simulink model "QPSK1"  (Simulink 8.2)
settings: Solver=ode45  StartTime=0.0  StopTime=10  MaxStep=0.00001  MinStep=0.000005  RelTol=1e-3
libraries: visionconversions x2, simulink_extras x2, dspsigops x2, commchan3 x1, commrandsrc2 x1, commsink2 x1, dspswit3 x1
settings Model: Creator=Yi_Liu  LastModifiedBy=Yi_Liu
settings DataIOCC: SignalLoggingSaveFormat=Dataset
settings OptimizationCC: ExpressionDepthLimit=128
settings DebuggingCC: FcnCallInpInsideContextMsg=EnableAllAsError  StateNameClashWarn=none
settings GRTTargetCC: CombineOutputUpdateFcns=on  GRTInterface=off

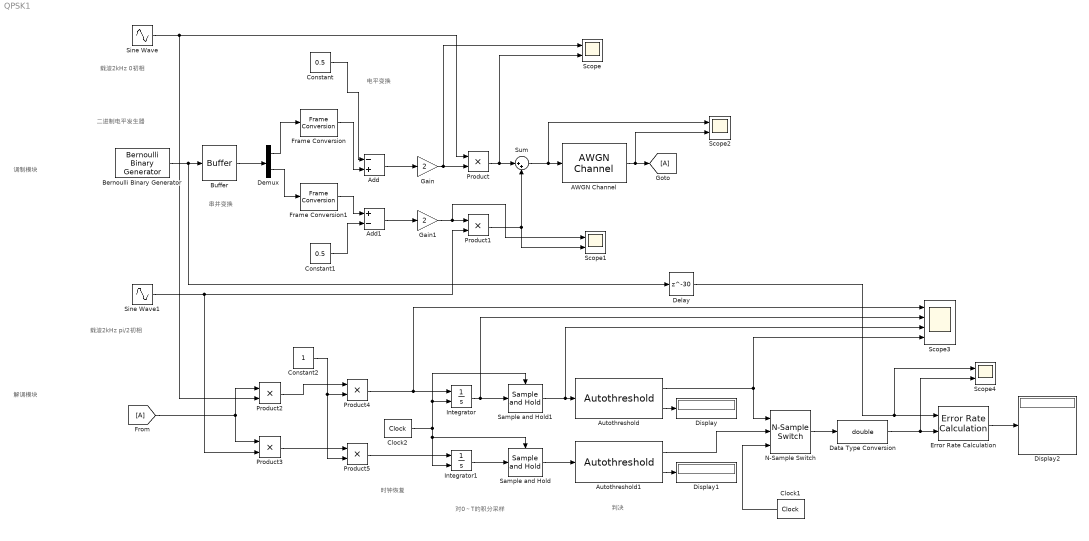
== system QPSK1 ==
  note: 判决
  note: 对0～T的积分采样
  note: 时钟恢复
  note: 调制模块
  note: 电平变换
  note: 串并变换
  note: 载波2kHz 0初相
  note: 二进制电平发生器
  note: 载波2kHz pi/2初相
  note: 解调模块
  AWGN Channel : commchan3/AWGN Channel  InputProcessing=Columns as channels (frame based)  seed=128  noiseMode=Variance from mask  EbNodB=10  EsNodB=10  SNRdB=10  bitsPerSym=1  Ps=1  Tsym=1  variance=0.01
  Add : Sum  Inputs=-+
  Add1 : Sum  Inputs=+-
  Autothreshold : visionconversions/Autothreshold  operator=>  threshOut=on  effMetricOut=off  userDefinedRange=off  umin=0  umax=255  outOfRngOpt=Warn and saturate  scaleThreshold=off  scaleFactor=1  P1Mode=Specify word length  P1WordLength=32  P1FracLength=30  P2Mode=Specify word length  P2WordLength=32  P2FracLength=22  P3Mode=Specify word length  P3WordLength=32  P3FracLength=14  P4Mode=Binary point scaling  P4WordLength=32  P4FracLength=15  Q1Mode=Specify word length  Q1WordLength=32  Q1FracLength=16  EMMode=Specify word length  EMWordLength=16  EMFracLength=14  roundingMode=Floor  overflowMode=off
  Autothreshold1 : visionconversions/Autothreshold  operator=>  threshOut=on  effMetricOut=off  userDefinedRange=off  umin=0  umax=255  outOfRngOpt=Warn and saturate  scaleThreshold=off  scaleFactor=1  P1Mode=Specify word length  P1WordLength=32  P1FracLength=30  P2Mode=Specify word length  P2WordLength=32  P2FracLength=22  P3Mode=Specify word length  P3WordLength=32  P3FracLength=14  P4Mode=Binary point scaling  P4WordLength=32  P4FracLength=15  Q1Mode=Specify word length  Q1WordLength=32  Q1FracLength=16  EMMode=Specify word length  EMWordLength=16  EMFracLength=14  roundingMode=Floor  overflowMode=off
  Bernoulli Binary Generator : commrandsrc2/Bernoulli Binary Generator  P=0.5  seed=64  Ts=0.001  frameBased=off  sampPerFrame=1  orient=off  outDataType=double
  Buffer : Buffer  N=2  TreatMby1Signals=One channel
  Clock1 : simulink_extras/Flip Flops/Clock  period=0.002
  Clock2 : simulink_extras/Flip Flops/Clock  period=0.002
  Constant : Constant  Value=0.5
  Constant1 : Constant  Value=0.5
  Constant2 : Constant
  Data Type Conversion : DataTypeConversion  OutDataTypeStr=double
  Delay : Delay  DelayLength=30  InitialCondition=0  SampleTime=0.0001
  Demux : Demux  Outputs=2
  Display : Display
  Display1 : Display
  Display2 : Display
  Error Rate Calculation : commsink2/Error Rate Calculation  N=0  st_delay=0  cp_mode=Entire frame  subframe=[]  PMode=Port  WsName=ErrorVec  RsMode2=off  stop=off  numErr=100  maxBits=1e6
  Frame Conversion : FrameConversion  OutFrame=Sample-based
  Frame Conversion1 : FrameConversion  OutFrame=Sample-based
  Gain : Gain  Gain=2
  Gain1 : Gain  Gain=2
  Integrator : Integrator  ExternalReset=rising
  Integrator1 : Integrator  ExternalReset=rising
  N-Sample Switch : dspswit3/N-Sample Switch  N=1  reset=on  TriggerType=Falling edge  Ts=-1
  Product{,1..5} (6 alike) : Product
  Sample and Hold : dspsigops/Sample and Hold  trig=Falling edge  initCond=0  latchinput=off
  Sample and Hold1 : dspsigops/Sample and Hold  trig=Falling edge  initCond=0  latchinput=off
  Scope{,1..2,4} (4 alike) : Scope  NumInputPorts=2
      Scope settings: YMin=-2~-2  YMax=2~2
      Scope1 settings: YMin=-2~-2  YMax=2~2
      Scope2 settings: YMin=-2~-2  YMax=2~2  SaveName=ScopeData2
      Scope4 settings: YMin=-2~-2  YMax=2~2  SaveName=ScopeData4
  Scope3 : Scope  NumInputPorts=4
      settings: YMin=-2~-2~-5~-5  YMax=2~2~5~5  SaveName=ScopeData3
  Sine Wave : Sin  Frequency=2*pi*2000  SampleTime=0
  Sine Wave1 : Sin  Frequency=2*pi*2000  Phase=pi/2  SampleTime=0
  Sum : Sum  Inputs=|++
  wires:
  Buffer/1 -> Demux/1
  Demux/1 -> Frame Conversion/1
  Demux/2 -> Frame Conversion1/1
  Add/1 -> Gain/1
  Frame Conversion1/1 -> Add1/1
  Frame Conversion/1 -> Add/2
  Constant/1 -> Add/1
  Constant1/1 -> Add1/2
  Add1/1 -> Gain1/1
  Gain1/1 -> Scope1/1, Product1/1
  Gain/1 -> Scope/1, Product/2
  Sine Wave1/1 -> Product1/2, Product3/2
  Sine Wave/1 -> Product2/2, Product/1
  Product1/1 -> Sum/2, Scope1/2
  Sum/1 -> Scope2/1, AWGN Channel/1
  AWGN Channel/1 -> Scope2/2, [A]
  Product3/1 -> Product5/1
  Constant2/1 -> Product4/2, Product5/2
  Clock2/1 -> Sample and Hold/Trigger, Integrator1/2, Integrator/2, Sample and Hold1/Trigger
  Product4/1 -> Scope3/1, Integrator/1
  Product5/1 -> Integrator1/1
  Autothreshold/1 -> Scope3/4, N-Sample Switch/1
  Autothreshold1/1 -> N-Sample Switch/2
  Clock1/1 -> N-Sample Switch/3
  Autothreshold/2 -> Display/1
  Autothreshold1/2 -> Display1/1
  [A] -> Product3/1, Product2/1
  Error Rate Calculation/1 -> Display2/1
  Product2/1 -> Product4/1
  Product/1 -> Scope/2, Sum/1
  Sample and Hold1/1 -> Scope3/3, Autothreshold/1
  Sample and Hold/1 -> Autothreshold1/1
  Integrator/1 -> Sample and Hold1/1, Scope3/2
  Integrator1/1 -> Sample and Hold/1
  Bernoulli Binary Generator/1 -> Delay/1, Buffer/1
  N-Sample Switch/1 -> Data Type Conversion/1
  Data Type Conversion/1 -> Scope4/2, Error Rate Calculation/2
  Delay/1 -> Scope4/1, Error Rate Calculation/1
